simulink library "simulink"  (R2014a)
settings: Solver=ode45  SolverMode=SingleTasking  StartTime=0.0  StopTime=10.0  RelTol=1e-3
PostLoadFcn:
  | setsysloc_simulink(bdroot)
undefined symbols (not defined in the file or in its folder): DiscIntNeverNeededParam, getdatatypespecs, NumBits1, NumBits2, sfunxy, sigbuilder_block, slcm, SlDemoSign, Slope1, Slope2
libraries: simulink x40, sl_helperblocks x2, eml_lib x1
(part 2 of 5)

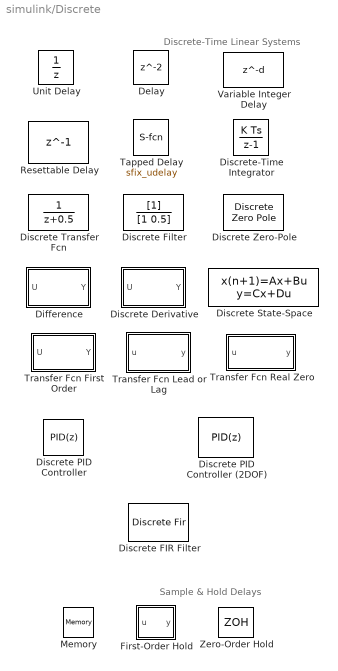
== system simulink/Discrete ==
  note: Sample & Hold Delays
  note: Discrete-Time Linear Systems
  Delay : Delay
  Difference : Subsystem  mask(Difference){ICPrevInput=0.0, InputProcessing=Inherited, OutMin=[], OutMax=[], OutDataTypeStr=Inherit: Inherit via internal rule, OutputDataTypeScalingMode=Inherit via internal rule, OutDataType=fixdt(1, 16), OutScaling=2^-10, LockScale=off, RndMeth=Floor, DoSatur=off}
      mask prompts: ICPrevInput "Simulink:masks:InitialConditionForPreviousInput_MP"; InputProcessing "Simulink:masks:InputProcessing_MP"; OutMin "Simulink:masks:OutputMinimum_MP"; OutMax "Simulink:masks:OutputMaximum_MP"; OutDataTypeStr "Simulink:masks:OutputDataType_MP"; OutputDataTypeScalingMode "Simulink:masks:OutputDataTypeMode_MP"; OutDataType "Simulink:masks:OutputDataTypeegFixdt116Fixdtsingle_MP"; OutScaling "Simulink:masks:OutputScalingSlopeEg29OrSlopeBias_MP"; LockScale "Simulink:masks:LockOutputDataTypeAgainstFxpTools_MP"; RndMeth "Simulink:masks:IntegerRoundingMode_MP"; DoSatur "Simulink:masks:SaturateToMaxOrMinWhenOverflowsOccur_MP"
      mask help: Simulink:masks:Difference_MD
      mask init:
      | blkH = gcbh;
      | blkName = getfullname(blkH);
      | 
      | set_param([blkName,'/Diff'], ...
      |     'RndMeth',RndMeth, ...
      | 	'DoSatur',DoSatur);
      | 
      | set_param([blkName,'/UD'], ...
      | 	'InputProcessing',InputProcessing);
      mask TypeOptions InputProcessing: Simulink:masks:ColumnsAsChannelsFrameBased | Simulink:masks:ElementsAsChannelsSampleBased | Simulink:masks:Inherited
      mask Callback OutDataTypeStr: fixptdialog(gcbh)
      mask TypeOptions OutputDataTypeScalingMode: double | single | int8 | uint8 | int16 | uint16 | int32 | uint32 | Specify via dialog | Inherit via internal rule | Inherit via back propagation
      mask Callback OutputDataTypeScalingMode: fixptdialog(gcbh)
      mask Callback OutDataType: fixptdialog(gcbh)
      mask TypeOptions RndMeth: Simulink:masks:Ceiling | Simulink:masks:Convergent | Simulink:masks:Floor | Simulink:masks:Nearest | Simulink:masks:Round | Simulink:masks:Simplest | Simulink:masks:Zero
      mask Display: dpoly([1 -1],[1 0],'z')
  Discrete Transfer Fcn : DiscreteTransferFcn
  Discrete Zero-Pole : DiscreteZeroPole  Poles=[0 0.5]  Gain=1
  Discrete Derivative : Subsystem  mask(Discrete Derivative){gainval=1.0, ICPrevScaledInput=0.0, InputProcessing=Inherited, OutMin=[], OutMax=[], OutDataTypeStr=Inherit: Inherit via internal rule, OutputDataTypeScalingMode=Inherit via internal rule, OutDataType=fixdt(1, 16), OutScaling=2^-10, LockScale=off, RndMeth=Floor, DoSatur=off}
      mask prompts: gainval "Simulink:masks:GainValue_MP"; ICPrevScaledInput "Simulink:masks:InitialConditionForPreviousWeightedInputKuTs_MP"; InputProcessing "Simulink:masks:InputProcessing_MP"; OutMin "Simulink:masks:OutputMinimum_MP"; OutMax "Simulink:masks:OutputMaximum_MP"; OutDataTypeStr "Simulink:masks:OutputDataType_MP"; OutputDataTypeScalingMode "Simulink:masks:OutputDataTypeMode_MP"; OutDataType "Simulink:masks:OutputDataTypeegFixdt116Fixdtsingle_MP"; OutScaling "Simulink:masks:OutputScalingSlopeEg29OrSlopeBias_MP"; LockScale "Simulink:masks:LockOutputDataTypeAgainstFxpTools_MP"; RndMeth "Simulink:masks:IntegerRoundingMode_MP"; DoSatur "Simulink:masks:SaturateToMaxOrMinWhenOverflowsOccur_MP"
      mask help: Simulink:masks:DiscreteDerivative_MD
      mask init:
      | blkH = gcbh;
      | blkName = getfullname(blkH);
      | 
      | if (gainval == 0.0)
      |     %avoid divide by zero warning
      |     inverseGainval = inf;
      | else
      |     inverseGainval = 1.0/double(gainval);
      | end
      | 
      | if isequal(OutDataTypeStr, 'Inherit: Inherit via internal rule')
      |     diffDT   = 'Inherit: Inherit via back propagation';
      |     tsampDT  = 'Inherit: Inherit via internal rule';
      |     tsampImp = 'Offline Scaling Adjustment';
      | else    
      |     diffDT   = OutDataTypeStr;
      |     tsampDT  = 'Inherit: Inherit via back propagation';
      |     tsampImp = 'Online Calculations';
      | end
      | 
      | if ~strcmp(get_param(bdroot(blkH),'SimulationStatus'), 'running')
      |     set_param([blkName,'/Diff'], ...
      |               'RndMeth',RndMeth, ...
      | 	          'DoSatur',DoSatur);
      |     set_param([blkName,'/TSamp'], ...
      |               'OutDataTypeStr',tsampDT, ...
      |               'RndMeth',RndMeth, ...
      |               'DoSatur',DoSatur, ...
      |               'TsampMathImp',tsampImp);
      | end
      | 
      | set_param([blkName,'/UD'], ...
      | 	'InputProcessing',InputProcessing);
      mask TypeOptions InputProcessing: Simulink:masks:ColumnsAsChannelsFrameBased | Simulink:masks:ElementsAsChannelsSampleBased | Simulink:masks:Inherited
      mask Callback OutDataTypeStr: fixptdialog(gcbh)
      mask TypeOptions OutputDataTypeScalingMode: double | single | int8 | uint8 | int16 | uint16 | int32 | uint32 | Specify via dialog | Inherit via internal rule | Inherit via back propagation
      mask Callback OutputDataTypeScalingMode: fixptdialog(gcbh)
      mask Callback OutDataType: fixptdialog(gcbh)
      mask TypeOptions RndMeth: Simulink:masks:Ceiling | Simulink:masks:Convergent | Simulink:masks:Floor | Simulink:masks:Nearest | Simulink:masks:Round | Simulink:masks:Simplest | Simulink:masks:Zero
      mask Display: text(0.5, 0.5, 'K (z-1)', 'horizontalAlignment', 'center', 'verticalAlignment', 'bottom');text(0.5, 0.5, 'Ts z', 'horizontalAlignment', 'center', 'verticalAlignment', 'top');plot([0.3 0.7],[0.5 0.5]);
  Discrete FIR Filter : DiscreteFir
  Discrete Filter : DiscreteFilter
  Discrete PID Controller : simulink/Continuous/PID Controller  Controller=PID  TimeDomain=Discrete-time  SampleTime=1  IntegratorMethod=Forward Euler  FilterMethod=Forward Euler  Form=Parallel  P=1  I=1  D=0  N=100  InitialConditionSource=internal  InitialConditionForIntegrator=0  InitialConditionForFilter=0  ExternalReset=none  LimitOutput=off  UpperSaturationLimit=inf  LowerSaturationLimit=-inf  LinearizeAsGain=off  AntiWindupMode=none  Kb=1  TrackingMode=off  Kt=1  PParamMin=[]  PParamMax=[]  IParamMin=[]  IParamMax=[]  DParamMin=[]  DParamMax=[]  NParamMin=[]  NParamMax=[]  KbParamMin=[]  KbParamMax=[]  KtParamMin=[]  KtParamMax=[]  POutMin=[]  POutMax=[]  IOutMin=[]  IOutMax=[]  DOutMin=[]  DOutMax=[]  NOutMin=[]  NOutMax=[]  KbOutMin=[]  KbOutMax=[]  KtOutMin=[]  KtOutMax=[]  IntegratorOutMin=[]  IntegratorOutMax=[]  FilterOutMin=[]  FilterOutMax=[]  SumOutMin=[]  SumOutMax=[]  SumI1OutMin=[]  SumI1OutMax=[]  SumI2OutMin=[]  SumI2OutMax=[]  SumI3OutMin=[]  SumI3OutMax=[]  SumDOutMin=[]  SumDOutMax=[]  SaturationOutMin=[]  SaturationOutMax=[]  IntegratorContinuousStateAttributes=''  IntegratorStateMustResolveToSignalObject=off  IntegratorRTWStateStorageClass=Auto  FilterContinuousStateAttributes=''  FilterStateMustResolveToSignalObject=off  FilterRTWStateStorageClass=Auto
  Discrete PID Controller (2DOF) : simulink/Continuous/PID Controller (2DOF)  Controller=PID  TimeDomain=Discrete-time  SampleTime=1  IntegratorMethod=Forward Euler  FilterMethod=Forward Euler  Form=Parallel  P=1  I=1  D=0  N=100  b=1  c=1  InitialConditionSource=internal  InitialConditionForIntegrator=0  InitialConditionForFilter=0  ExternalReset=none  LimitOutput=off  UpperSaturationLimit=inf  LowerSaturationLimit=-inf  LinearizeAsGain=off  AntiWindupMode=none  Kb=1  TrackingMode=off  Kt=1  PParamMin=[]  PParamMax=[]  IParamMin=[]  IParamMax=[]  DParamMin=[]  DParamMax=[]  NParamMin=[]  NParamMax=[]  bParamMin=[]  bParamMax=[]  cParamMin=[]  cParamMax=[]  KbParamMin=[]  KbParamMax=[]  KtParamMin=[]  KtParamMax=[]  POutMin=[]  POutMax=[]  IOutMin=[]  IOutMax=[]  DOutMin=[]  DOutMax=[]  NOutMin=[]  NOutMax=[]  bOutMin=[]  bOutMax=[]  cOutMin=[]  cOutMax=[]  KbOutMin=[]  KbOutMax=[]  KtOutMin=[]  KtOutMax=[]  IntegratorOutMin=[]  IntegratorOutMax=[]  FilterOutMin=[]  FilterOutMax=[]  SumOutMin=[]  SumOutMax=[]  Sum1OutMin=[]  Sum1OutMax=[]  Sum2OutMin=[]  Sum2OutMax=[]  Sum3OutMin=[]  Sum3OutMax=[]  SumI1OutMin=[]  SumI1OutMax=[]  SumI2OutMin=[]  SumI2OutMax=[]  SumI3OutMin=[]  SumI3OutMax=[]  SumDOutMin=[]  SumDOutMax=[]  SaturationOutMin=[]  SaturationOutMax=[]  IntegratorContinuousStateAttributes=''  IntegratorStateMustResolveToSignalObject=off  IntegratorRTWStateStorageClass=Auto  FilterContinuousStateAttributes=''  FilterStateMustResolveToSignalObject=off  FilterRTWStateStorageClass=Auto
  Discrete State-Space : DiscreteStateSpace
  Discrete-Time Integrator : DiscreteIntegrator  ICPrevOutput=DiscIntNeverNeededParam  ICPrevScaledInput=DiscIntNeverNeededParam
  First-Order Hold : Subsystem  DisableCoverage=on  mask(First-Order Hold){Ts=1}
      mask prompts: Ts "Simulink:masks:SampleTime_MP"
      mask help: Simulink:masks:FirstOrderHold_MD
      mask Help: This block implements a first-order hold by extrapolating between sample points using a first-order polynomial.
      mask Display: plot(0,0,100,100,[90,70,50,30,10],[60,40,80,30,20])
  Memory : Memory
  Resettable Delay : Delay  DelayLength=1  InitialConditionSource=Input port  ExternalReset=Rising
      settings: InputPortMap=u0,r5,p4
  Tapped Delay : S-Function  FunctionName=sfix_udelay  Parameters=samptime,vinit,NumDelays,NumDelays,DelayOrder,includeCurrent,3  EnableBusSupport=off  mask(Tapped Delay Line){vinit=0.0, samptime=-1, NumDelays=4, DelayOrder=Oldest, includeCurrent=off}
      mask prompts: vinit "Simulink:masks:InitialCondition_MP"; samptime "Simulink:masks:SampleTime_MP"; NumDelays "Simulink:masks:NumberOfDelays_MP"; DelayOrder "Simulink:masks:OrderOutputVectorStartingWith_MP"; includeCurrent "Simulink:masks:IncludeCurrentInputInOutputVector_MP"
      mask help: Simulink:masks:TappedDelayLine_MD
      mask init:
      | if isempty(NumDelays)
      |    NumDelays = 1;
      | end
      mask TypeOptions DelayOrder: Simulink:masks:Oldest | Simulink:masks:Newest
      mask Display: fprintf(' %d\nDelays\n',(NumDelays))
  Transfer Fcn First Order : Subsystem  mask(First Order Transfer Fcn){PoleZ=0.95, ICPrevOutput=0.0, RndMeth=Floor, DoSatur=off}
      mask prompts: PoleZ "Simulink:masks:PoleinZPlane_MP"; ICPrevOutput "Simulink:masks:InitialConditionForPreviousOutput_MP"; RndMeth "Simulink:masks:IntegerRoundingMode_MP"; DoSatur "Simulink:masks:SaturateToMaxOrMinWhenOverflowsOccur_MP"
      mask help: Simulink:masks:FirstOrderTransferFcn_MD
      mask init:
      | blkH = gcbh;
      | blkName = getfullname(blkH);
      | 
      | vRndMeth = get_param(blkH,'RndMeth');
      | vDoSatur = get_param(blkH,'DoSatur');
      | 
      | set_param([blkName,'/Gain'],'RndMeth',vRndMeth, ...
      | 	'DoSatur',vDoSatur);
      | set_param([blkName,'/Diff'],'RndMeth',vRndMeth, ...
      | 	'DoSatur',vDoSatur);
      | set_param([blkName,'/Sum'],'RndMeth',vRndMeth, ...
      | 	'DoSatur',vDoSatur);
      mask TypeOptions RndMeth: Simulink:masks:Ceiling | Simulink:masks:Convergent | Simulink:masks:Floor | Simulink:masks:Nearest | Simulink:masks:Round | Simulink:masks:Simplest | Simulink:masks:Zero
      mask Display: dpoly([1-PoleZ 0],[1 -PoleZ],'z')
  Transfer Fcn Lead or Lag : Subsystem  mask(Lead or Lag Compensator){PoleZ=0.95, ZeroZ=0.75, ICPrevOutput=0.0, ICPrevInput=0.0, RndMeth=Floor, DoSatur=off}
      mask prompts: PoleZ "Simulink:masks:PoleOfCompensatorinZPlane_MP"; ZeroZ "Simulink:masks:ZeroOfCompensatorinZPlane_MP"; ICPrevOutput "Simulink:masks:InitialConditionForPreviousOutput_MP"; ICPrevInput "Simulink:masks:InitialConditionForPreviousInput_MP"; RndMeth "Simulink:masks:IntegerRoundingMode_MP"; DoSatur "Simulink:masks:SaturateToMaxOrMinWhenOverflowsOccur_MP"
      mask help: Simulink:masks:LeadOrLagCompensator_MD
      mask init:
      | if ((PoleZ < 0) || (PoleZ >= 1))
      |    error('Pole position must be a positive number less than 1')
      | end
      | if ((ZeroZ < 0) || (ZeroZ > 1))
      |    error('Zero position must be a positive number less than or equal to 1')
      | end
      | blkH = gcbh;
      | blkName = getfullname(blkH);
      | 
      | vRndMeth = get_param(blkH,'RndMeth');
      | vDoSatur = get_param(blkH,'DoSatur');
      | DCGain = (1-ZeroZ)./(1-PoleZ);
      | maxGain = max( 1, max(max(abs(DCGain))) );
      | OutputSlopeMult = 2^ceil(log2(maxGain));
      | set_param([blkName,'/GainZero'],'RndMeth',vRndMeth, ...
      | 	'DoSatur',vDoSatur);
      | set_param([blkName,'/GainPole'],'RndMeth',vRndMeth, ...
      | 	'DoSatur',vDoSatur);
      | set_param([blkName,'/Downcast'],'RndMeth',vRndMeth, ...
      | 	'DoSatur',vDoSatur);
      | set_param([blkName,'/Sum'],'RndMeth',vRndMeth, ...
      | 	'DoSatur',vDoSatur);
      mask TypeOptions RndMeth: Simulink:masks:Ceiling | Simulink:masks:Convergent | Simulink:masks:Floor | Simulink:masks:Nearest | Simulink:masks:Round | Simulink:masks:Simplest | Simulink:masks:Zero
      mask Display: dpoly([1 -ZeroZ],[1 -PoleZ],'z')
  Transfer Fcn Real Zero : Subsystem  mask(Transfer Fcn Real Zero){ZeroZ=0.75, ICPrevInput=0.0, InputProcessing=Inherited, RndMeth=Floor, DoSatur=off}
      mask prompts: ZeroZ "Simulink:masks:ZeroinZPlane_MP"; ICPrevInput "Simulink:masks:InitialConditionForPreviousInput_MP"; InputProcessing "Simulink:masks:InputProcessing_MP"; RndMeth "Simulink:masks:IntegerRoundingMode_MP"; DoSatur "Simulink:masks:SaturateToMaxOrMinWhenOverflowsOccur_MP"
      mask help: Simulink:masks:TransferFcnRealZero_MD
      mask init:
      | blkH = gcbh;
      | blkName = getfullname(blkH);
      | 
      | vRndMeth = get_param(blkH,'RndMeth');
      | vDoSatur = get_param(blkH,'DoSatur');
      | DCGain = (1-ZeroZ);
      | maxGain = max( 1, max(max(abs(DCGain))) );
      | OutputSlopeMult = 2^ceil(log2(maxGain));
      | set_param([blkName,'/GainZero'],'RndMeth',vRndMeth, ...
      | 	'DoSatur',vDoSatur);
      | set_param([blkName,'/Sum'],'RndMeth',vRndMeth, ...
      | 	'DoSatur',vDoSatur);
      | set_param([blkName,'/Delay Input'], ...
      | 	'InputProcessing',InputProcessing);
      mask TypeOptions InputProcessing: Simulink:masks:ColumnsAsChannelsFrameBased | Simulink:masks:ElementsAsChannelsSampleBased | Simulink:masks:Inherited
      mask TypeOptions RndMeth: Simulink:masks:Ceiling | Simulink:masks:Convergent | Simulink:masks:Floor | Simulink:masks:Nearest | Simulink:masks:Round | Simulink:masks:Simplest | Simulink:masks:Zero
      mask Display: dpoly([1 -ZeroZ],[1 0],'z')
  Unit Delay : UnitDelay  SampleTime=-1
  Variable Integer Delay : Delay  DelayLengthSource=Input port
      settings: InputPortMap=u0,p1
  Zero-Order Hold : ZeroOrderHold

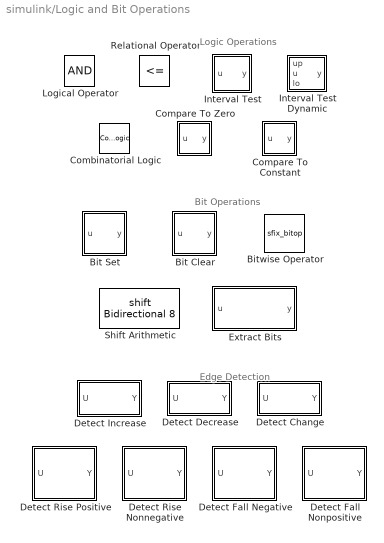
== system simulink/Logic and Bit Operations ==
  note: Edge Detection
  note: Logic Operations
  note: Bit Operations
  Bit Clear : Subsystem  mask(Bit Clear){iBit=0}
      mask prompts: iBit "Simulink:masks:IndexOfBit0IsLeastSignificant_MP"
      mask help: Simulink:masks:BitClear_MD
      mask init:
      | if length(iBit) == 1
      |   dispStr = sprintf('Clear\nbit %d',double(iBit));
      | else
      |   dispStr=sprintf('Vector\nBit Clear');
      | end
      mask Display: disp(dispStr)
  Bit Set : Subsystem  mask(Bit Set){iBit=0}
      mask prompts: iBit "Simulink:masks:IndexOfBit0IsLeastSignificant_MP"
      mask help: Simulink:masks:BitSet_MD
      mask init:
      | if length(iBit) == 1
      |   dispStr = sprintf('Set\nbit %d',double(iBit));
      | else
      |   dispStr=sprintf('Vector\nBit Set');
      | end
      mask Display: disp(dispStr)
  Bitwise Operator : S-Function  FunctionName=sfix_bitop  Parameters=UseBitMask,NumInputPorts,BitMask,BitMaskRealWorld,logicop  EnableBusSupport=off  mask(Bitwise Operator){logicop=AND, UseBitMask=on, NumInputPorts=1, BitMask=bin2dec('11011001'), BitMaskRealWorld=Stored Integer}
      mask prompts: logicop "Simulink:masks:Operator_MP"; UseBitMask "Simulink:masks:UseBitMask_MP"; NumInputPorts "Simulink:masks:NumberOfInputPorts_MP"; BitMask "Simulink:masks:BitMask_MP"; BitMaskRealWorld "Simulink:masks:TreatMaskAs_MP"
      mask help: Simulink:masks:BitwiseOperator_MD
      mask init:
      | str = '';
      | if UseBitMask
      |   [m,n] = size(BitMask);
      |   if ischar(BitMask)
      |     len = m;
      |     n = 1;
      |   else
      |     len = m * n;
      |   end
      |   internalBitMask = zeros(m,n);
      |   if isnumeric(BitMask)
      |     if ~isreal(BitMask)
      |       error(DAStudio.message('Simulink:blocks:BitMaskNotComplex'));
      |     end
      |     for i=1:len,
      |       internalBitMask(i) = BitMask(i);
      |     end
      |   elseif ischar(BitMask)
      |     for i=1:m,
      |       internalBitMask(i) = hex2dec(BitMask(i,:));
      |     end
      |   elseif iscell(BitMask)
      |     for i=1:len,
      |       if isnumeric( BitMask{i} )
      |         internalBitMask(i) = BitMask{i};
      |       elseif ischar( BitMask{i} )
      |         internalBitMask(i) = hex2dec(BitMask{i});
      |       else
      |         errordlg(['Data type is not supported at cell item ', num2str(i) ]);
      |       end
      |     end
      |   end
      |   BitMask = internalBitMask;
      |   for i=1:len
      |     if BitMask(i) > (2^52)-1
      |       error(DAStudio.message('Simulink:blocks:BitMaskWordLengthTooLarge')); 
      |     end
      |   end 
      |   if len == 1
      |      if BitMaskRealWorld == 1 || BitMask(1) < 0
      |        str=num2str(BitMask(1));
      |      else
      |        str=['0x',dec2hex(floor(BitMask(1)))];
      |      end
      |   else
      |      str='Masks';
      |   end
      | else
      |   BitMask = 0;
      |   str='';
      | end
      mask TypeOptions logicop: Simulink:masks:AND | Simulink:masks:OR | Simulink:masks:NAND | Simulink:masks:NOR | Simulink:masks:XOR | Simulink:masks:NOT
      mask Callback logicop: fixptdialog(gcbh)
      mask Callback UseBitMask: fixptdialog(gcbh)
      mask TypeOptions BitMaskRealWorld: Simulink:masks:RealWorldValue | Simulink:masks:StoredInteger
      mask Display: fprintf(['Bitwise\n',logicop,'\n',str])
  Combinatorial Logic : CombinatorialLogic
  Compare To Constant : Subsystem  mask(Compare To Constant){relop=<=, const=3.0, OutDataTypeStr=boolean, ZeroCross=on}
      mask prompts: relop "Simulink:masks:Operator_MP"; const "Simulink:masks:ConstantValue_MP"; OutDataTypeStr "Simulink:masks:OutputDataType_MP"; ZeroCross "Simulink:masks:EnableZerocrossingDetection_MP"
      mask help: Simulink:masks:CompareToConstant_MD
      mask init:
      | blkName = gcb;
      | 
      | if strcmp(get_param(gcbh,'OutDataTypeStr'),'boolean')
      | 	setValue = 'boolean';
      | else
      | 	setValue = 'fixdt(0, 8)';
      | end
      | 
      | set_param([blkName,'/Compare'],'relop',relop, ...
      | 	'OutDataTypeStr', setValue, 'ZeroCross', ZeroCross);
      | 
      | str = [relop,' C']; %default
      | const_str = strtrim(get_param(blkName, 'const'));
      | 
      | if isempty(const)
      |     % Expression could not be successfully evaluated during edit time
      |     str = [relop, ' ', const_str];
      | else
      |     if length(const) == 1 
      |         if Simulink.data.isSupportedEnumClass(class(const))
      |         % Special Handling for Enumerations
      |             if Simulink.data.getEnumTypeInfo(class(const), 'AddClassNameToEnumNames')
      |                 str = [relop, ' ', const_str];
      |             else
      |                 str = [relop, ' ', char(const)];
      |             end
      |         elseif(isfloat(const) || isinteger(const)) 
      |             str = [relop, ' ', num2str(const)];
      |         end
      |     end
      | end
      mask TypeOptions relop: == | ~= | < | <= | >= | >
      mask TypeOptions OutDataTypeStr: Simulink:masks:uint8 | Simulink:masks:boolean
      mask Callback ZeroCross: sl('zeroCrossEnable', gcbh);
      mask Display: disp(str)
  Compare To Zero : Subsystem  mask(Compare To Zero){relop=<=, OutDataTypeStr=boolean, ZeroCross=on}
      mask prompts: relop "Simulink:masks:Operator_MP"; OutDataTypeStr "Simulink:masks:OutputDataType_MP"; ZeroCross "Simulink:masks:EnableZerocrossingDetection_MP"
      mask help: Simulink:masks:CompareToZero_MD
      mask init:
      | blkName = gcb;
      | 
      | if strcmp(get_param(gcbh,'OutDataTypeStr'),'boolean')
      | 	setValue = 'boolean';
      | else
      |     setValue = 'fixdt(0, 8)';
      | end
      | 
      | set_param([blkName,'/Compare'],'relop',relop, ...
      | 	'OutDataTypeStr', setValue, 'ZeroCross', ZeroCross);
      mask TypeOptions relop: == | ~= | < | <= | >= | >
      mask TypeOptions OutDataTypeStr: Simulink:masks:uint8 | Simulink:masks:boolean
      mask Callback ZeroCross: sl('zeroCrossEnable', gcbh);
      mask Display: disp([relop,' 0'])
  Detect Change : Subsystem  mask(Detect Change){vinit=0, InputProcessing=Inherited, OutDataTypeStr=boolean}
      mask prompts: vinit "Simulink:masks:InitialCondition_MP"; InputProcessing "Simulink:masks:InputProcessing_MP"; OutDataTypeStr "Simulink:masks:OutputDataType_MP"
      mask help: Simulink:masks:DetectChange_MD
      mask init:
      | initDetectBlocks();
      mask TypeOptions InputProcessing: Simulink:masks:ColumnsAsChannelsFrameBased | Simulink:masks:ElementsAsChannelsSampleBased | Simulink:masks:Inherited
      mask TypeOptions OutDataTypeStr: Simulink:masks:uint8 | Simulink:masks:boolean
      mask Display: fprintf('U ~= U/z')
  Detect Decrease : Subsystem  mask(Detect Decrease){vinit=0.0, InputProcessing=Inherited, OutDataTypeStr=boolean}
      mask prompts: vinit "Simulink:masks:InitialCondition_MP"; InputProcessing "Simulink:masks:InputProcessing_MP"; OutDataTypeStr "Simulink:masks:OutputDataType_MP"
      mask help: Simulink:masks:DetectDecrease_MD
      mask init:
      | initDetectBlocks();
      mask TypeOptions InputProcessing: Simulink:masks:ColumnsAsChannelsFrameBased | Simulink:masks:ElementsAsChannelsSampleBased | Simulink:masks:Inherited
      mask TypeOptions OutDataTypeStr: Simulink:masks:uint8 | Simulink:masks:boolean
      mask Display: fprintf('U < U/z')
  Detect Increase : Subsystem  mask(Detect Increase){vinit=0.0, InputProcessing=Inherited, OutDataTypeStr=boolean}
      mask prompts: vinit "Simulink:masks:InitialCondition_MP"; InputProcessing "Simulink:masks:InputProcessing_MP"; OutDataTypeStr "Simulink:masks:OutputDataType_MP"
      mask help: Simulink:masks:DetectIncrease_MD
      mask init:
      | initDetectBlocks();
      mask TypeOptions InputProcessing: Simulink:masks:ColumnsAsChannelsFrameBased | Simulink:masks:ElementsAsChannelsSampleBased | Simulink:masks:Inherited
      mask TypeOptions OutDataTypeStr: Simulink:masks:uint8 | Simulink:masks:boolean
      mask Display: fprintf('U > U/z')
  Detect Fall Negative : Subsystem  mask(Detect Fall Negative){vinit=0, InputProcessing=Inherited, OutDataTypeStr=boolean}
      mask prompts: vinit "Simulink:masks:InitialCondition_MP"; InputProcessing "Simulink:masks:InputProcessing_MP"; OutDataTypeStr "Simulink:masks:OutputDataType_MP"
      mask help: Simulink:masks:DetectFallNegative_MD
      mask init:
      | vinit=double(vinit);
      | 
      | initDetectBlocks();
      mask TypeOptions InputProcessing: Simulink:masks:ColumnsAsChannelsFrameBased | Simulink:masks:ElementsAsChannelsSampleBased | Simulink:masks:Inherited
      mask TypeOptions OutDataTypeStr: Simulink:masks:uint8 | Simulink:masks:boolean
      mask Display: fprintf('U < 0\n&  NOT\nU/z < 0')
  Detect Fall Nonpositive : Subsystem  mask(Detect Fall Nonpositive){vinit=0, InputProcessing=Inherited, OutDataTypeStr=boolean}
      mask prompts: vinit "Simulink:masks:InitialCondition_MP"; InputProcessing "Simulink:masks:InputProcessing_MP"; OutDataTypeStr "Simulink:masks:OutputDataType_MP"
      mask help: Simulink:masks:DetectFallNonpositive_MD
      mask init:
      | vinit=double(vinit);
      | 
      | initDetectBlocks();
      mask TypeOptions InputProcessing: Simulink:masks:ColumnsAsChannelsFrameBased | Simulink:masks:ElementsAsChannelsSampleBased | Simulink:masks:Inherited
      mask TypeOptions OutDataTypeStr: Simulink:masks:uint8 | Simulink:masks:boolean
      mask Display: fprintf('U <= 0\n&  NOT\nU/z <= 0')
  Detect Rise Nonnegative : Subsystem  mask(Detect Rise Nonnegative){vinit=0, InputProcessing=Inherited, OutDataTypeStr=boolean}
      mask prompts: vinit "Simulink:masks:InitialCondition_MP"; InputProcessing "Simulink:masks:InputProcessing_MP"; OutDataTypeStr "Simulink:masks:OutputDataType_MP"
      mask help: Simulink:masks:DetectRiseNonnegative_MD
      mask init:
      | vinit=double(vinit);
      | 
      | initDetectBlocks();
      mask TypeOptions InputProcessing: Simulink:masks:ColumnsAsChannelsFrameBased | Simulink:masks:ElementsAsChannelsSampleBased | Simulink:masks:Inherited
      mask TypeOptions OutDataTypeStr: Simulink:masks:uint8 | Simulink:masks:boolean
      mask Display: fprintf('U >= 0\n&  NOT\nU/z >= 0')
  Detect Rise Positive : Subsystem  mask(Detect Rise Positive){vinit=0, InputProcessing=Inherited, OutDataTypeStr=boolean}
      mask prompts: vinit "Simulink:masks:InitialCondition_MP"; InputProcessing "Simulink:masks:InputProcessing_MP"; OutDataTypeStr "Simulink:masks:OutputDataType_MP"
      mask help: Simulink:masks:DetectRisePositive_MD
      mask init:
      | vinit=double(vinit);
      | 
      | initDetectBlocks();
      mask TypeOptions InputProcessing: Simulink:masks:ColumnsAsChannelsFrameBased | Simulink:masks:ElementsAsChannelsSampleBased | Simulink:masks:Inherited
      mask TypeOptions OutDataTypeStr: Simulink:masks:uint8 | Simulink:masks:boolean
      mask Display: fprintf('U > 0\n&  NOT\nU/z > 0')
  Extract Bits : Subsystem  mask(Extract Bits){bitsToExtract=Upper half, numBits=8, bitIdxRange=[0 7], outScalingMode=Preserve fixed-point scaling}
      mask prompts: bitsToExtract "Simulink:masks:BitsToExtract_MP"; numBits "Simulink:masks:NumberOfBits_MP"; bitIdxRange "Simulink:masks:BitIndicesstartEnd0basedRelativeToLSB_MP"; outScalingMode "Simulink:masks:OutputScalingMode_MP"
      mask help: Simulink:masks:ExtractBits_MD
      mask init:
      | str = fixpt_extractbits_mask('icon', numBits, bitIdxRange); 
      | fixpt_extractbits_mask_script;
      mask TypeOptions bitsToExtract: Simulink:masks:UpperHalf | Simulink:masks:LowerHalf | Simulink:masks:RangeStartingWithMostSignificantBit | Simulink:masks:RangeEndingWithLeastSignificantBit | Simulink:masks:RangeOfBits
      mask Callback bitsToExtract: fixpt_extractbits_mask;
      mask TypeOptions outScalingMode: Simulink:masks:PreserveFixedPointScaling | Simulink:masks:TreatBitFieldAsAnInteger
      mask Display: disp(str);
  Interval Test : Subsystem  mask(Interval Test){IntervalClosedRight=on, uplimit=0.5, IntervalClosedLeft=on, lowlimit=-0.5, OutDataTypeStr=boolean}
      mask prompts: IntervalClosedRight "Simulink:masks:IntervalClosedOnRight_MP"; uplimit "Simulink:masks:UpperLimit_MP"; IntervalClosedLeft "Simulink:masks:IntervalClosedOnLeft_MP"; lowlimit "Simulink:masks:LowerLimit_MP"; OutDataTypeStr "Simulink:masks:OutputDataType_MP"
      mask help: Simulink:masks:IntervalTest_MD
      mask init:
      | if IntervalClosedLeft
      |   lOff = 0;
      |   lRelop = '<=';
      | else
      |   lOff = 0.1;
      |   lRelop = '<';
      | end
      | if IntervalClosedRight
      |   rOff = 0;
      |   uRelop = '<=';
      | else
      |   rOff = 0.1;
      |   uRelop = '<';
      | end
      | 
      | blkH = gcbh;
      | blkName = getfullname(blkH);
      | 
      | set_param([blkName,'/Upper Test'],'relop',uRelop);
      | set_param([blkName,'/Lower Test'],'relop',lRelop);
      | if strcmp(get_param(blkH,'OutDataTypeStr'),'boolean')
      | set_param([blkName,'/AND'],'OutDataTypeStr','boolean');
      | else
      | set_param([blkName,'/AND'],'OutDataTypeStr','fixdt(0, 8)');
      | end
      mask TypeOptions OutDataTypeStr: Simulink:masks:uint8 | Simulink:masks:boolean
      mask Display: plot([0 1],[0.3 0.3],[0.3 0.3],[0 1],[0 0.2 0.2],[0.35 0.35 0.55-lOff],[0.2 0.2 0.55 0.55],[0.55+lOff 0.75 0.75 0.55+rOff],[0.55 0.55 1],[0.55-rOff 0.35 0.35]);
  Interval Test Dynamic : Subsystem  mask(Interval Test Dynamic){IntervalClosedRight=on, IntervalClosedLeft=on, OutDataTypeStr=boolean}
      mask prompts: IntervalClosedRight "Simulink:masks:IntervalClosedOnRight_MP"; IntervalClosedLeft "Simulink:masks:IntervalClosedOnLeft_MP"; OutDataTypeStr "Simulink:masks:OutputDataType_MP"
      mask help: Simulink:masks:IntervalTest_MD
      mask init:
      | if IntervalClosedLeft
      |   lOff = 0;
      |   lRelop = '<=';
      | else
      |   lOff = 0.1;
      |   lRelop = '<';
      | end
      | if IntervalClosedRight
      |   rOff = 0;
      |   uRelop = '<=';
      | else
      |   rOff = 0.1;
      |   uRelop = '<';
      | end
      | blkH = gcbh;
      | blkName = getfullname(gcbh);
      | 
      | set_param([blkName,'/Upper Test'],'relop',uRelop);
      | set_param([blkName,'/Lower Test'],'relop',lRelop);
      | if strcmp(get_param(blkH,'OutDataTypeStr'),'boolean')
      | set_param([blkName,'/FixPt Logical Operator'],'OutDataTypeStr','boolean');
      | else
      | set_param([blkName,'/FixPt Logical Operator'],'OutDataTypeStr','fixdt(0, 8)');
      | end
      mask TypeOptions OutDataTypeStr: Simulink:masks:uint8 | Simulink:masks:boolean
      mask Display: plot(0.35+0.65*[0 1],[0.3 0.3],0.35+0.65*[0.3 0.3],[0 1],0.35+0.65*[0 0.2 0.2],[0.35 0.35 0.55-lOff],0.35+0.65*[0.2 0.2 0.55 0.55],[0.55+lOff 0.75 0.75 0.55+rOff],0.35+0.65*[0.55 0.55 1],[0.55-rOff 0.35 0.35]);
  Logical Operator : Logic  AllPortsSameDT=off  OutDataTypeStr=boolean
  Relational Operator : RelationalOperator  Operator=<=  OutDataTypeStr=boolean
  Shift Arithmetic : ArithShift  BitShiftNumber=8

== system simulink/Lookup Tables ==
  note: Lookup Tables
  1-D Lookup Table : Lookup_n-D  NumberOfTableDimensions=1  BreakpointsForDimension1=[-5:5]  Table=tanh([-5:5])  InternalRulePriority=Speed  RndMeth=Simplest  InputSameDT=on
  2-D Lookup Table : Lookup_n-D  BreakpointsForDimension1=[1:3]  BreakpointsForDimension2=[1:3]  InternalRulePriority=Speed  RndMeth=Simplest  InputSameDT=on
  Cosine : Subsystem  mask(Sine and Cosine){Formula=cos(2*pi*u), NumDataPoints=(2^5)+1, OutputWordLength=16, InternalRulePriority=Speed}
      mask prompts: Formula "Simulink:masks:OutputFormula_MP"; NumDataPoints "Simulink:masks:NumberOfDataPointsForLookupTable_MP"; OutputWordLength "Simulink:masks:OutputWordLength_MP"; InternalRulePriority "Simulink:masks:InternalRulePriorityForLookupTable_MP"
      mask help: Simulink:masks:SineAndCosine_MD
      mask init:
      | if (~isnumeric(OutputWordLength)) || ( length(OutputWordLength) > 1 ) || ( OutputWordLength < 2 ) || ( floor(OutputWordLength) ~= OutputWordLength )
      |     error(DAStudio.message('Simulink:blocks:SineLookupWordLengthTooSmall'));
      | end
      | if (~isnumeric(NumDataPoints)) || ( length(NumDataPoints) > 1 ) || ( NumDataPoints < 2 ) || ( floor(NumDataPoints) ~= NumDataPoints )
      |     error(DAStudio.message('Simulink:blocks:SineLookupNumDataPtsTooSmall'));
      | end
      | if ( 2^(OutputWordLength-2) + 1 ) < NumDataPoints
      |     smallEnoughNumDataPoints = ( 2^(OutputWordLength-2) + 1 );
      |     bigEnoughOutputWordLength = ceil(log2(NumDataPoints-1))+2;
      |     error(DAStudio.message('Simulink:blocks:SineLookupEitherTooSmall',...
      |         NumDataPoints, ...
      |         smallEnoughNumDataPoints, ...
      |         OutputWordLength, ...
      |         bigEnoughOutputWordLength));
      | end
      | slsincos(Formula);
      mask TypeOptions Formula: Simulink:masks:sin2PiU | Simulink:masks:cos2PiU | Simulink:masks:expj2PiU | Simulink:masks:sincos2PiU
      mask TypeOptions InternalRulePriority: Simulink:masks:InternalRulePrioritySpeed | Simulink:masks:InternalRulePriorityPrecision
  Direct Lookup Table (n-D) : LookupNDDirect
  Interpolation Using Prelookup : Interpolation_n-D  InternalRulePriority=Speed
  Lookup Table Dynamic : S-Function  FunctionName=sfix_look1_dyn  Parameters=OutputDataTypeScalingMode,(getdatatypespecs(OutDataType,OutScaling,DblOver,0, 0, OutputDataTypeScalingMode)),[DoSatur RndMeth-1],DblOver,dolog,LookUpMeth  EnableBusSupport=off  mask(Lookup Table Dynamic){LookUpMeth=Interpolation-Use End Values, OutDataTypeStr=double, OutputDataTypeScalingMode=Specify via dialog, OutDataType=fixdt('double'), OutScaling=2^-10, LockScale=off, RndMeth=Floor, DoSatur=off}
      mask prompts: LookUpMeth "Simulink:masks:LookupMethod_MP"; OutDataTypeStr "Simulink:masks:OutputDataType_MP"; OutputDataTypeScalingMode "Simulink:masks:OutputDataTypeMode_MP"; OutDataType "Simulink:masks:OutputDataTypeegFixdt116Fixdtsingle_MP"; OutScaling "Simulink:masks:OutputScalingSlopeEg29OrSlopeBias_MP"; LockScale "Simulink:masks:LockOutputDataTypeAgainstFxpTools_MP"; RndMeth "Simulink:masks:IntegerRoundingMode_MP"; DoSatur "Simulink:masks:SaturateToMaxOrMinWhenOverflowsOccur_MP"
      mask help: Simulink:masks:LookupTableDynamic_MD
      mask init:
      | DblOver = 0;
      | dolog = 0;
      mask TypeOptions LookUpMeth: Simulink:masks:InterpolationExtrapolation | Simulink:masks:InterpolationUseEndValues | Simulink:masks:UseInputNearest | Simulink:masks:UseInputBelow | Simulink:masks:UseInputAbove
      mask Callback OutDataTypeStr: fixptdialog(gcbh)
      mask TypeOptions OutputDataTypeScalingMode: Specify via dialog | Inherit via back propagation
      mask Callback OutputDataTypeScalingMode: fixptdialog(gcbh)
      mask Callback OutDataType: fixptdialog(gcbh)
      mask TypeOptions RndMeth: Simulink:masks:Ceiling | Simulink:masks:Convergent | Simulink:masks:Floor | Simulink:masks:Nearest | Simulink:masks:Round | Simulink:masks:Simplest | Simulink:masks:Zero
      mask Display:
      | port_label('Input',1,'x');
      | port_label('Input',2,'xdat');
      | port_label('Input',3,'ydat');
      | port_label('Output',1,'y');
  Prelookup : PreLookup  BreakpointsData=[10:10:110]  ExtrapMethod=Linear
  Sine : Subsystem  mask(Sine and Cosine){Formula=sin(2*pi*u), NumDataPoints=(2^5)+1, OutputWordLength=16, InternalRulePriority=Speed}
      mask prompts: Formula "Simulink:masks:OutputFormula_MP"; NumDataPoints "Simulink:masks:NumberOfDataPointsForLookupTable_MP"; OutputWordLength "Simulink:masks:OutputWordLength_MP"; InternalRulePriority "Simulink:masks:InternalRulePriorityForLookupTable_MP"
      mask help: Simulink:masks:SineAndCosine_MD
      mask init: same as simulink/Lookup Tables/Cosine
      mask TypeOptions Formula: Simulink:masks:sin2PiU | Simulink:masks:cos2PiU | Simulink:masks:expj2PiU | Simulink:masks:sincos2PiU
      mask TypeOptions InternalRulePriority: Simulink:masks:InternalRulePrioritySpeed | Simulink:masks:InternalRulePriorityPrecision
  n-D Lookup Table : Lookup_n-D  NumberOfTableDimensions=3  BreakpointsForDimension3=[5, 7]  Table=reshape(repmat([4 5 6;16 19 20;10 18 23],1,2),[3,3,2])  InternalRulePriority=Speed  RndMeth=Simplest  InputSameDT=on
  wires:
  Prelookup/1 -> Interpolation Using Prelookup/1
  Prelookup/2 -> Interpolation Using Prelookup/2

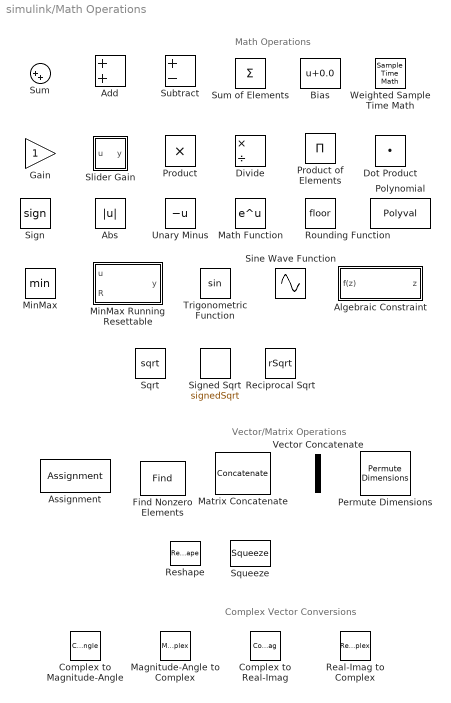
== system simulink/Math Operations ==
  note: Vector/Matrix Operations
  note: Math Operations
  note: Complex Vector Conversions
  Abs : Abs
  Add : Sum
  Algebraic Constraint : Subsystem  mask(Algebraic Constraint){z0=0}
      mask prompts: z0 "Simulink:masks:InitialGuess_MP"
      mask help: Simulink:masks:AlgebraicConstraint_MD
      mask Help:
      | This block outputs the value necessary to produce a zero at the input. The output must affect the input through some feedback path. This allows you to specify algebraic equations for index 1 differential/algebraic systems (DAE's).
      | 
      | By default, the initial guess is zero.  You can improve the efficiency of the algebraic loop solver by providing an initial guess that is close to the solution value.
      mask Display: disp('Solve\nf(z) = 0')
  Assignment : Assignment  DiagnosticForDimensions=Warning
  Bias : Bias  Bias=0.0
  Complex to Magnitude-Angle : ComplexToMagnitudeAngle
  Complex to Real-Imag : ComplexToRealImag
  Divide : Product  Inputs=*/
  Dot Product : DotProduct  InputSameDT=on  OutDataTypeStr=Inherit: Inherit via internal rule
  Find Nonzero Elements : Find  NumberOfInputDimensions=3  IndexMode=Zero-based
  Gain : Gain
  Magnitude-Angle to Complex : MagnitudeAngleToComplex
  Math Function : Math  SaturateOnIntegerOverflow=on
  Matrix Concatenate : Concatenate  Mode=Multidimensional array  ConcatenateDimension=2
  MinMax : MinMax
  MinMax Running Resettable : Subsystem  mask(MinMax Running Resettable){Function=min, vinit=0.0}
      mask prompts: Function "Simulink:masks:Function_MP"; vinit "Simulink:masks:InitialCondition_MP"
      mask help: Simulink:masks:MinMaxRunningResettable_MD
      mask init:
      | dim = size(vinit);
      | if (length(dim) > 2) || (min(dim) ~= 1)
      |     error('The parameter ''Initial condition'' must be a vector or a scalar');
      |     return;
      | else
      |    set_param([gcb,'/MinMax'],'Function',get_param(gcbh,'Function'));
      | end
      mask TypeOptions Function: Simulink:masks:min | Simulink:masks:max
      mask Display: disp([char((Function==1)*'min'+(Function==2)*'max'),'(u,y)'])
  Permute Dimensions : PermuteDimensions
  Polynomial : Polyval  Coefs=[ +2.081618890e-019, -1.441693666e-014, +4.719686976e-010, -8.536869453e-006, +1.621573104e-001, -8.087801117e+001 ]
  Product : Product
  Product of Elements : Product  Inputs=*
  Real-Imag to Complex : RealImagToComplex
  Reciprocal Sqrt : Sqrt  Operator=rSqrt  SaturateOnIntegerOverflow=on
  Reshape : Reshape
  Rounding Function : Rounding
  Sign : Signum
  Signed Sqrt : Sqrt  Operator=signedSqrt  SaturateOnIntegerOverflow=on
  Sine Wave Function : Sin  TimeSource=Use external signal  SampleTime=0
  Slider Gain : Subsystem  LoadFcn=slideg Load  StartFcn=slideg StartFcn  StopFcn=slideg StopFcn  mask(Slider Gain){low=0, gain=1, high=2}
      mask prompts: low "Simulink:masks:Low_MP"; gain "Simulink:masks:Gain_MP"; high "Simulink:masks:High_MP"
      settings: CopyFcn=slideg Copy  DeleteFcn=slideg DeleteBlock  NameChangeFcn=slideg NameChange  OpenFcn=slideg Open  CloseFcn=slideg Close  ParentCloseFcn=slideg ParentClose
      mask Display: disp(gain)
  Sqrt : Sqrt  SaturateOnIntegerOverflow=on
  Squeeze : Squeeze
  Subtract : Sum  Inputs=+-
  Sum : Sum  Inputs=|++
      settings: CopyFcn=set_param(gcbh,'ShowName','off','CopyFcn','')
  Sum of Elements : Sum  Inputs=+
  Trigonometric Function : Trigonometry
  Unary Minus : UnaryMinus
  Vector Concatenate : Concatenate
  Weighted Sample Time Math : SampleTimeMath

== system simulink/Model Verification ==
  note: Run-time Model Verification
  Assertion : Assertion
  Check Discrete Gradient : Subsystem  Description=| du / dt | < 1  mask(Checks_Gradient){gradient=1, enabled=on, callback=, stopWhenAssertionFail=on, export=off, icon=graphic}
      mask prompts: gradient "Simulink:masks:MaximumGradient_MP"; enabled "Simulink:masks:EnableAssertion_MP"; callback "Simulink:masks:SimulationCallbackWhenAssertionFails_MP"; stopWhenAssertionFail "Simulink:masks:StopSimulationWhenAssertionFails_MP"; export "Simulink:masks:OutputAssertionSignal_MP"; icon "Simulink:masks:SelectIconType_MP"
      mask help: Simulink:masks:Checks_Gradient_MD
      mask init:
      | update_assert_sys(gcbh);
      mask Callback enabled: update_assert_sys(gcbh,'updateSimulationCallBackEditField');
      mask TypeOptions icon: Simulink:masks:graphic | Simulink:masks:text
      mask Display: image(imread('Checks_Gradient.bmp','bmp'),'center')
  Check Dynamic Gap : Subsystem  Description=sig < min || max < sig  mask(Checks_DGap){enabled=on, callback=, stopWhenAssertionFail=on, export=off, icon=graphic}
      mask prompts: enabled "Simulink:masks:EnableAssertion_MP"; callback "Simulink:masks:SimulationCallbackWhenAssertionFails_MP"; stopWhenAssertionFail "Simulink:masks:StopSimulationWhenAssertionFails_MP"; export "Simulink:masks:OutputAssertionSignal_MP"; icon "Simulink:masks:SelectIconType_MP"
      mask help: Simulink:masks:Checks_DGap_MD
      mask init:
      | update_assert_sys(gcbh);
      mask Callback enabled: update_assert_sys(gcbh,'updateSimulationCallBackEditField');
      mask TypeOptions icon: Simulink:masks:graphic | Simulink:masks:text
      mask Display:
      | port_label('input', 1, 'max');
      | port_label('input', 2, 'min');
      | port_label('input', 3, 'sig');
      | image(imread('Checks_DGap.bmp','bmp'),'center')
  Check Dynamic Range : Subsystem  Description=min < sig < max  mask(Checks_DRange){enabled=on, callback=, stopWhenAssertionFail=on, export=off, icon=graphic}
      mask prompts: enabled "Simulink:masks:EnableAssertion_MP"; callback "Simulink:masks:SimulationCallbackWhenAssertionFails_MP"; stopWhenAssertionFail "Simulink:masks:StopSimulationWhenAssertionFails_MP"; export "Simulink:masks:OutputAssertionSignal_MP"; icon "Simulink:masks:SelectIconType_MP"
      mask help: Simulink:masks:Checks_DRange_MD
      mask init:
      | update_assert_sys(gcbh);
      mask Callback enabled: update_assert_sys(gcbh,'updateSimulationCallBackEditField');
      mask TypeOptions icon: Simulink:masks:graphic | Simulink:masks:text
      mask Display:
      | port_label('input', 1,'max');
      | port_label('input', 2, 'min');
      | port_label('input', 3, 'sig');
      | image(imread('Checks_DRange.bmp','bmp'),'center')
  Check Static Gap : Subsystem  Description=u <= 0 || 100 <= u  mask(Checks_SGap){max=100, max_included=on, min=0, min_included=on, enabled=on, callback=, stopWhenAssertionFail=on, export=off, icon=graphic}
      mask prompts: max "Simulink:masks:UpperBound_MP"; max_included "Simulink:masks:InclusiveUpperBound_MP"; min "Simulink:masks:LowerBound_MP"; min_included "Simulink:masks:InclusiveLowerBound_MP"; enabled "Simulink:masks:EnableAssertion_MP"; callback "Simulink:masks:SimulationCallbackWhenAssertionFails_MP"; stopWhenAssertionFail "Simulink:masks:StopSimulationWhenAssertionFails_MP"; export "Simulink:masks:OutputAssertionSignal_MP"; icon "Simulink:masks:SelectIconType_MP"
      mask help: Simulink:masks:Checks_SGap_MD
      mask init:
      | update_assert_sys(gcbh);
      mask Callback enabled: update_assert_sys(gcbh,'updateSimulationCallBackEditField');
      mask TypeOptions icon: Simulink:masks:graphic | Simulink:masks:text
      mask Display: image(imread('Checks_SGap.bmp','bmp'),'center')
  Check Static Range : Subsystem  Description=0 <= u <= 100  mask(Checks_SRange){max=100, max_included=on, min=0, min_included=on, enabled=on, callback=, stopWhenAssertionFail=on, export=off, icon=graphic}
      mask prompts: max "Simulink:masks:UpperBound_MP"; max_included "Simulink:masks:InclusiveUpperBound_MP"; min "Simulink:masks:LowerBound_MP"; min_included "Simulink:masks:InclusiveLowerBound_MP"; enabled "Simulink:masks:EnableAssertion_MP"; callback "Simulink:masks:SimulationCallbackWhenAssertionFails_MP"; stopWhenAssertionFail "Simulink:masks:StopSimulationWhenAssertionFails_MP"; export "Simulink:masks:OutputAssertionSignal_MP"; icon "Simulink:masks:SelectIconType_MP"
      mask help: Simulink:masks:Checks_SRange_MD
      mask init:
      | update_assert_sys(gcbh);
      mask Callback enabled: update_assert_sys(gcbh,'updateSimulationCallBackEditField');
      mask TypeOptions icon: Simulink:masks:graphic | Simulink:masks:text
      mask Display: image(imread('Checks_SRange.bmp','bmp'),'center')
  Check Dynamic Lower Bound : Subsystem  Description=min < sig  mask(Checks_DMin){Enabled=on, callback=, stopWhenAssertionFail=on, export=off, icon=graphic}
      mask prompts: Enabled "Simulink:masks:EnableAssertion_MP"; callback "Simulink:masks:SimulationCallbackWhenAssertionFails_MP"; stopWhenAssertionFail "Simulink:masks:StopSimulationWhenAssertionFails_MP"; export "Simulink:masks:OutputAssertionSignal_MP"; icon "Simulink:masks:SelectIconType_MP"
      mask help: Simulink:masks:Checks_DMin_MD
      mask init:
      | update_assert_sys(gcbh);
      mask Callback Enabled: update_assert_sys(gcbh,'updateSimulationCallBackEditField');
      mask TypeOptions icon: Simulink:masks:graphic | Simulink:masks:text
      mask Display:
      | port_label('input', 1,'min');
      | port_label('input', 2, 'sig');
      | image(imread('Checks_DMin.bmp','bmp'),'center')
  Check Dynamic Upper Bound : Subsystem  Description=sig < max  mask(Checks_DMax){enabled=on, callback=, stopWhenAssertionFail=on, export=off, icon=graphic}
      mask prompts: enabled "Simulink:masks:EnableAssertion_MP"; callback "Simulink:masks:SimulationCallbackWhenAssertionFails_MP"; stopWhenAssertionFail "Simulink:masks:StopSimulationWhenAssertionFails_MP"; export "Simulink:masks:OutputAssertionSignal_MP"; icon "Simulink:masks:SelectIconType_MP"
      mask help: Simulink:masks:Checks_DMax_MD
      mask init:
      | update_assert_sys(gcbh);
      mask Callback enabled: update_assert_sys(gcbh,'updateSimulationCallBackEditField');
      mask TypeOptions icon: Simulink:masks:graphic | Simulink:masks:text
      mask Display:
      | port_label('input', 1,'max');
      | port_label('input', 2, 'sig');
      | image(imread('Checks_DMax.bmp','bmp'),'center')
  Check Input Resolution : Subsystem  Description=-Inf < u < +Inf  mask(Checks_Resolution){resolution=1, enabled=on, callback=, stopWhenAssertionFail=on, export=off}
      mask prompts: resolution "Simulink:masks:Resolution_MP"; enabled "Simulink:masks:EnableAssertion_MP"; callback "Simulink:masks:SimulationCallbackWhenAssertionFails_MP"; stopWhenAssertionFail "Simulink:masks:StopSimulationWhenAssertionFails_MP"; export "Simulink:masks:OutputAssertionSignal_MP"
      mask help: Simulink:masks:Checks_Resolution_MD
      mask init:
      | update_assert_sys(gcbh, length(resolution));
      mask Callback enabled: update_assert_sys(gcbh,'updateSimulationCallBackEditField');
      mask Display: image(imread('Checks_Resolution.bmp','bmp'),'center')
  Check Static Lower Bound : Subsystem  Description=0 <= u  mask(Checks_SMin){min=0, min_included=on, enabled=on, callback=, stopWhenAssertionFail=on, export=off, icon=graphic}
      mask prompts: min "Simulink:masks:LowerBound_MP"; min_included "Simulink:masks:InclusiveBoundary_MP"; enabled "Simulink:masks:EnableAssertion_MP"; callback "Simulink:masks:SimulationCallbackWhenAssertionFails_MP"; stopWhenAssertionFail "Simulink:masks:StopSimulationWhenAssertionFails_MP"; export "Simulink:masks:OutputAssertionSignal_MP"; icon "Simulink:masks:SelectIconType_MP"
      mask help: Simulink:masks:Checks_SMin_MD
      mask init:
      | update_assert_sys(gcbh);
      mask Callback enabled: update_assert_sys(gcbh, 'updateSimulationCallBackEditField');
      mask TypeOptions icon: Simulink:masks:graphic | Simulink:masks:text
      mask Display: image(imread('Checks_SMin.bmp','bmp'),'center')
  Check Static Upper Bound : Subsystem  Description=u <= 0  mask(Checks_SMax){max=0, max_included=on, enabled=on, callback=, stopWhenAssertionFail=on, export=off, icon=graphic}
      mask prompts: max "Simulink:masks:UpperBound_MP"; max_included "Simulink:masks:InclusiveBoundary_MP"; enabled "Simulink:masks:EnableAssertion_MP"; callback "Simulink:masks:SimulationCallbackWhenAssertionFails_MP"; stopWhenAssertionFail "Simulink:masks:StopSimulationWhenAssertionFails_MP"; export "Simulink:masks:OutputAssertionSignal_MP"; icon "Simulink:masks:SelectIconType_MP"
      mask help: Simulink:masks:Checks_SMax_MD
      mask init:
      | update_assert_sys(gcbh);
      mask Callback enabled: update_assert_sys(gcbh,'updateSimulationCallBackEditField');
      mask TypeOptions icon: Simulink:masks:graphic | Simulink:masks:text
      mask Display: image(imread('Checks_SMax.bmp','bmp'),'center')
